simulink model "mdl_4reac_idealpump_growth"  (R2020b)
settings: Solver=VariableStepAuto  StartTime=0.0  StopTime=1000  FixedStep=h  MaxStep=1  RelTol=1e-3  AbsTol=1e-6
undefined symbols (not defined in the file): p
settings Model: Creator=nobel  LastModifiedBy=natha

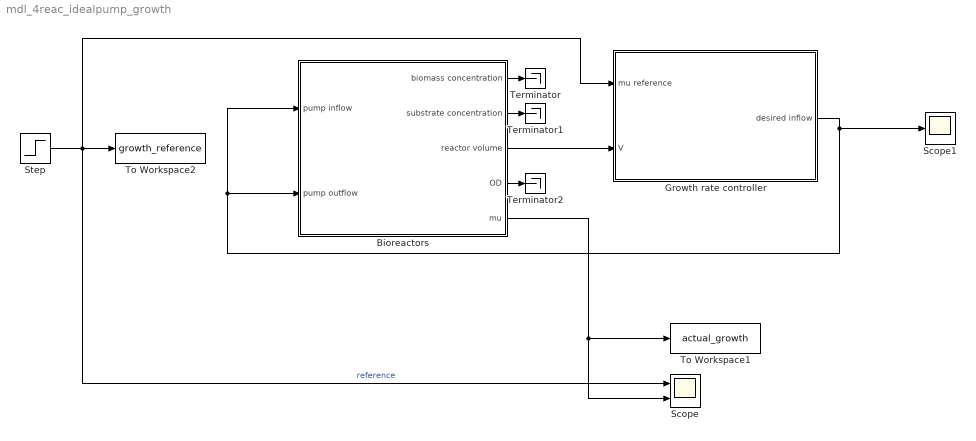
== system mdl_4reac_idealpump_growth ==
  Bioreactors : Subsystem  mask{p=p}
      mask prompts: p "Reactor Parameter Struct"
  Growth rate controller : Subsystem  mask{p=p}
      mask prompts: p "Reactor Parameter Struct"
  Scope : Scope  NumInputPorts=2
  Scope1 : Scope
  Step : Step  Time=p.growth_rate.step_time  Before=p.growth_rate.init_val  After=p.growth_rate.final_val  SampleTime=0
  Terminator : Terminator
  Terminator1 : Terminator
  Terminator2 : Terminator
  To Workspace1 : ToWorkspace  VariableName=actual_growth  SampleTime=-1
  To Workspace2 : ToWorkspace  VariableName=growth_reference  SampleTime=-1
  wires:
  Step/1 -> Scope/1, Growth rate controller/1(mu reference), To Workspace2/1  "reference"
  Bioreactors/2(substrate concentration) -> Terminator1/1
  Bioreactors/5(mu) -> To Workspace1/1, Scope/2
  Bioreactors/1(biomass concentration) -> Terminator/1
  Growth rate controller/1(desired inflow) -> Bioreactors/2(pump outflow), Bioreactors/1(pump inflow), Scope1/1
  Bioreactors/3(reactor volume) -> Growth rate controller/2(V)
  Bioreactors/4(OD) -> Terminator2/1

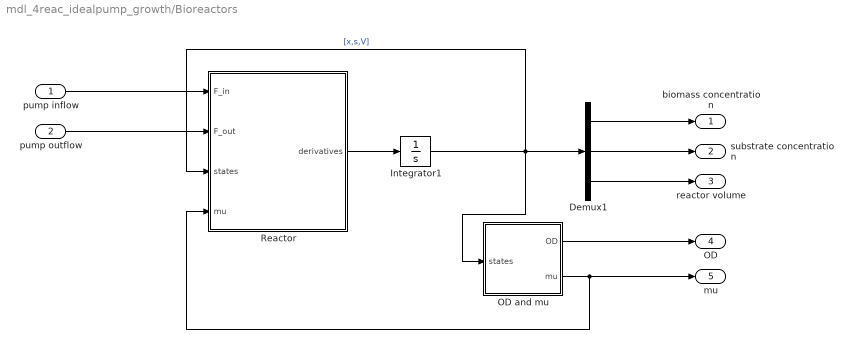
== system mdl_4reac_idealpump_growth/Bioreactors ==
  pump inflow : Inport
  pump outflow : Inport  Port=2
  Demux1 : Demux  Outputs=3
  Integrator1 : Integrator  InitialCondition=[p.init_x; p.init_s; p.init_v];
  OD and mu : MATLAB Function  TreatAsAtomicUnit=on
  Reactor : MATLAB Function  TreatAsAtomicUnit=on
  biomass concentration : Outport
  substrate concentration : Outport  Port=2
  reactor volume : Outport  Port=3
  OD : Outport  Port=4
  mu : Outport  Port=5
  wires:
  pump inflow/1 -> Reactor/1(F_in)
  Demux1/3 -> reactor volume/1
  pump outflow/1 -> Reactor/2(F_out)
  Reactor/1(derivatives) -> Integrator1/1
  OD and mu/2(mu) -> Reactor/4(mu), mu/1
  OD and mu/1(OD) -> OD/1
  Demux1/2 -> substrate concentration/1
  Demux1/1 -> biomass concentration/1
  Integrator1/1 -> Reactor/3(states), Demux1/1, OD and mu/1(states)  "[x,s,V]"

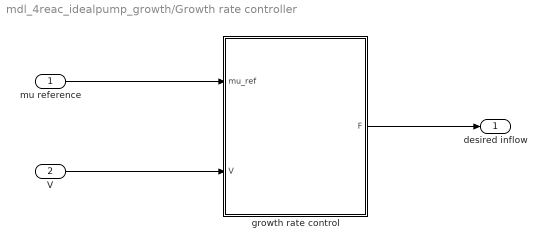
== system mdl_4reac_idealpump_growth/Growth rate controller ==
  mu reference : Inport
  V : Inport  Port=2
  growth rate control : MATLAB Function  TreatAsAtomicUnit=on
  desired inflow : Outport
  wires:
  mu reference/1 -> growth rate control/1(mu_ref)
  V/1 -> growth rate control/2(V)
  growth rate control/1(F) -> desired inflow/1

== matlab function mdl_4reac_idealpump_growth/Bioreactors/Reactor ==
  data: F_in input; derivatives output size=3*p.num_reac; F_out input; states input; mu input; p parameter
function derivatives   = fcn(F_in,F_out,states, mu, p)

x=states(1:p.num_reac);
s=states(p.num_reac+(1:p.num_reac));
V=states(2*p.num_reac+(1:p.num_reac));

D = F_in./V;

%dx    (Concentration of biomass in the biorreactor)
dx= mu.*x - D.*x;

%ds    (Concentration of substrate in the biorreactor)
ds= -p.y.*mu.*x + D.*(p.s_f - s);

%dV    (Volume of liquid inside the biorreactor)
dV= F_in - F_out;


derivatives = [dx; ds; dV];

== matlab function mdl_4reac_idealpump_growth/Bioreactors/OD and mu ==
  data: states input; OD output; mu output; p parameter
function [OD,mu] = fcn(states, p)

x=states(1:p.num_reac);
s=states(p.num_reac+(1:p.num_reac));
V=states(2*p.num_reac+(1:p.num_reac));

OD=x./p.m_p./p.nOD;
mu = p.mu_max.*s./(p.K_s+s);

== matlab function mdl_4reac_idealpump_growth/Growth rate controller/growth rate control ==
  data: mu_ref input; V input; F output
function F = fcn(mu_ref,V)

F = mu_ref.*V;
